simulink model "Phase2_Section4_observer"  (R2021b)
settings: Solver=VariableStepAuto  StartTime=0.0  StopTime=50.0  RelTol=1e-3
values from neighbouring files (symbols this model uses):
  A = [0 1 0; 244.86 -0.094 -26.29; 0 0 -250]    [Phase2_Section1.m]    (also in Phase2_Section2.m; Phase2_Section3.m; Phase2_Section4.m; Phase2_Section5.m)
  Ahat_slow = A - L_slow * C    [Phase2_Section4.m]
  B = [0; 0; 5]    [Phase2_Section1.m]    (also in Phase2_Section2.m; Phase2_Section3.m; Phase2_Section4.m; Phase2_Section5.m)
  C = [1 0 0]    [Phase2_Section1.m]    (also in Phase2_Section2.m; Phase2_Section3.m; Phase2_Section4.m; Phase2_Section5.m)
  K1 = place(A, B, p_fast)    [Phase2_Section1.m]    (also in Phase2_Section2.m; Phase2_Section3.m; Phase2_Section4.m = place(A, B, [-4 -2 -3]); Phase2_Section5.m = place(A, B, [-4 -2 -3]))
  L_slow = transpose(K_slow)    [Phase2_Section4.m]
settings Model: Creator=odeut  LastModifiedBy=odeut

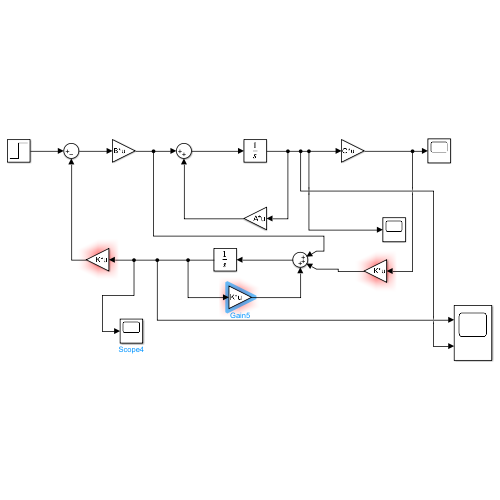
[thumbnail: Simulink's stored preview of the top-level diagram]
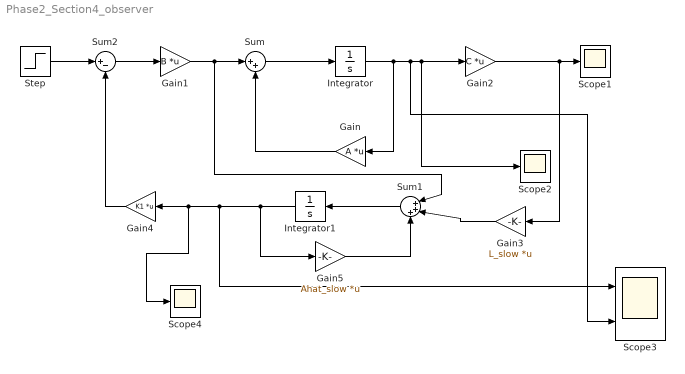
== system Phase2_Section4_observer ==
  Gain : Gain  Gain=A  Multiplication=Matrix(K*u)
  Gain1 : Gain  Gain=B  Multiplication=Matrix(K*u)
  Gain2 : Gain  Gain=C  Multiplication=Matrix(K*u)
  Gain3 : Gain  Gain=L_slow  Multiplication=Matrix(K*u)
  Gain4 : Gain  Gain=K1  Multiplication=Matrix(K*u)
  Gain5 : Gain  Gain=Ahat_slow  Multiplication=Matrix(K*u)
  Integrator : Integrator
  Integrator1 : Integrator
  Scope1 : Scope
  Scope2 : Scope
  Scope3 : Scope  NumInputPorts=2
  Scope4 : Scope
  Step : Step  SampleTime=0
  Sum : Sum  Inputs=|++
  Sum1 : Sum  Inputs=|+++
  Sum2 : Sum  Inputs=|+-
  wires:
  Gain4/1 -> Sum2/2
  Gain/1 -> Sum/2
  Integrator1/1 -> Gain5/1, Scope3/1, Scope4/1, Gain4/1
  Gain3/1 -> Sum1/2
  Sum1/1 -> Integrator1/1
  Step/1 -> Sum2/1
  Integrator/1 -> Scope3/2, Scope2/1, Gain2/1, Gain/1
  Gain1/1 -> Sum1/1, Sum/1
  Gain2/1 -> Scope1/1, Gain3/1
  Sum2/1 -> Gain1/1
  Sum/1 -> Integrator/1
  Gain5/1 -> Sum1/3
